simulink model "mmn_kart_candidate1_hdl"  (R2025a)
settings: Solver=FixedStepDiscrete  StartTime=0.0  StopTime=30  FixedStep=5e-5  RelTol=1e-3
undefined symbols (not defined in the file): ampa_decay, current_gain, gaba_decay, leakage_gain, refractory
libraries: simulink x3
settings Model: DataTypeOverride=Off  MinMaxOverflowLogging=MinMaxAndOverflow  FPTShortcutValueString='{{},{''BaselineRun'',1,1,1,''BaselineRun'','''',{},''M'',''SD'',''''}}'  Creator=PC  LastModifiedBy=PC
settings OptimizationCC: BlockReduction=off  ConditionallyExecuteInputs=off  DefaultParameterBehavior=Inlined
settings DebuggingCC: SingleTaskRateTransMsg=error

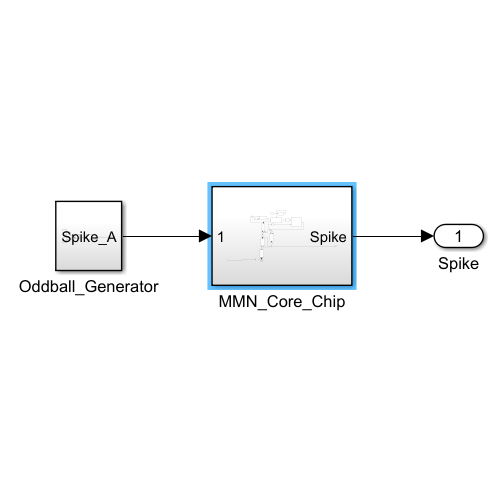
[thumbnail: Simulink's stored preview of the top-level diagram]
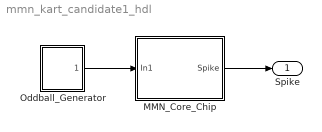
== system mmn_kart_candidate1_hdl ==
  MMN_Core_Chip : Subsystem
  Oddball_Generator : Subsystem
  Spike : Outport
  wires:
  Oddball_Generator/1(Spike_A) -> MMN_Core_Chip/1(In1)
  MMN_Core_Chip/1(Spike) -> Spike/1

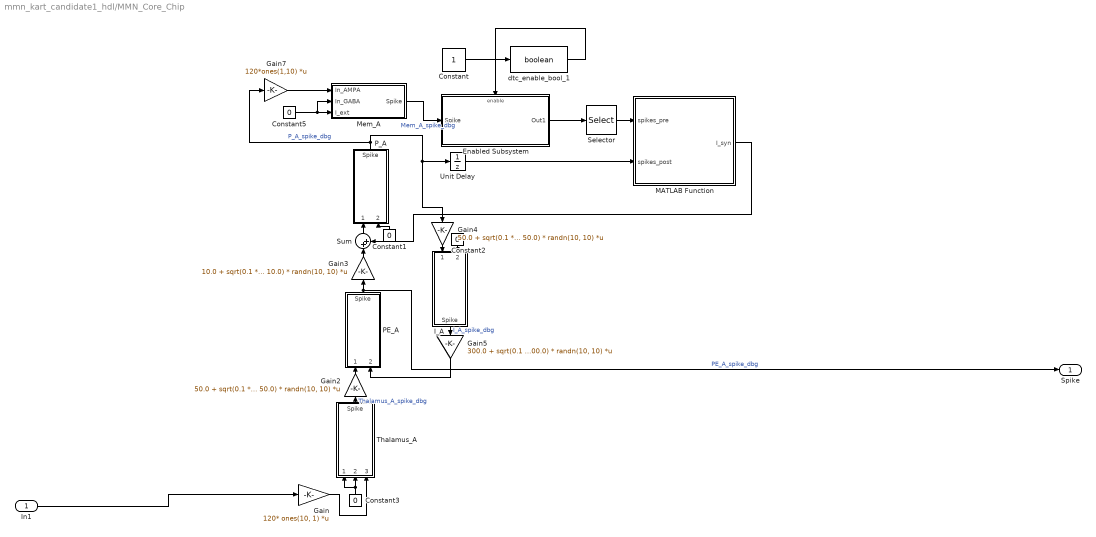
== system mmn_kart_candidate1_hdl/MMN_Core_Chip ==
  In1 : Inport  OutDataTypeStr=boolean  SampleTime=5e-5
  Constant : Constant  OutDataTypeStr=fixdt(1,24,8)  SampleTime=5e-5
  Constant{1..3,5} (4 alike) : Constant  Value=0  OutDataTypeStr=fixdt(1,24,8)
  Enabled Subsystem : Subsystem  TreatAsAtomicUnit=on
  Gain : Gain  Gain=120* ones(10, 1)  Multiplication=Matrix(K*u)  ParamDataTypeStr=fixdt(1,24,8)  OutDataTypeStr=fixdt(1,24,8)  SaturateOnIntegerOverflow=on
  Gain2 : Gain  Gain=50.0 + sqrt(0.1 * 50.0) * randn(10, 10)  Multiplication=Matrix(K*u)  ParamDataTypeStr=fixdt(1,24,8)  OutDataTypeStr=fixdt(1,24,8)  SaturateOnIntegerOverflow=on
  Gain3 : Gain  Gain=10.0 + sqrt(0.1 * 10.0) * randn(10, 10)  Multiplication=Matrix(K*u)  ParamDataTypeStr=fixdt(1,24,8)  OutDataTypeStr=fixdt(1,24,8)  SaturateOnIntegerOverflow=on
  Gain4 : Gain  Gain=50.0 + sqrt(0.1 * 50.0) * randn(10, 10)  Multiplication=Matrix(K*u)  ParamDataTypeStr=fixdt(1,24,8)  OutDataTypeStr=fixdt(1,24,8)  SaturateOnIntegerOverflow=on
  Gain5 : Gain  Gain=300.0 + sqrt(0.1 * 300.0) * randn(10, 10)  Multiplication=Matrix(K*u)  ParamDataTypeStr=fixdt(1,24,8)  OutDataTypeStr=fixdt(1,24,8)  SaturateOnIntegerOverflow=on
  Gain7 : Gain  Gain=120*ones(1,10)  Multiplication=Matrix(K*u)  ParamDataTypeStr=fixdt(1,24,8)  OutDataTypeStr=fixdt(1,24,8)  SaturateOnIntegerOverflow=on
  I_A : Subsystem
  MATLAB Function : MATLAB Function  TreatAsAtomicUnit=on  SystemSampleTime=5e-5
  Mem_A : Subsystem
  PE_A : Subsystem
  P_A : Subsystem
  Selector : Selector  InputPortWidth=12000  IndexOptions=Index vector (dialog)  Indices=[1:120:12000]  OutputSizes=1
  Sum : Sum  Inputs=|++  OutDataTypeStr=fixdt(1,24,8)  AccumDataTypeStr=fixdt(1,24,8)  SaturateOnIntegerOverflow=on
  Thalamus_A : Subsystem
  Unit Delay : UnitDelay  SampleTime=-1  HasFrameUpgradeWarning=on
  dtc_enable_bool_1 : DataTypeConversion  OutDataTypeStr=boolean  RndMeth=Floor
  Spike : Outport  OutDataTypeStr=boolean
  wires:
  Constant5/1 -> Mem_A/2("In_GABA "), Mem_A/3(I_ext)
  Sum/1 -> P_A/1(In_AMPA)
  Constant3/1 -> Thalamus_A/1(In_AMPA), Thalamus_A/2("In_GABA ")
  Constant2/1 -> I_A/2("In_GABA ")
  MATLAB Function/1(I_syn) -> Sum/2
  In1/1 -> Gain/1
  Enabled Subsystem/1(Out1) -> Selector/1
  Unit Delay/1 -> MATLAB Function/2(spikes_post)
  Mem_A/1(Spike) -> Enabled Subsystem/1(Spike)  "Mem_A_spike_dbg"
  Constant1/1 -> P_A/2("In_GABA ")
  Gain3/1 -> Sum/1
  Gain5/1 -> PE_A/2("In_GABA ")
  Gain4/1 -> I_A/1(In_AMPA)
  Gain7/1 -> Mem_A/1(In_AMPA)
  Gain2/1 -> PE_A/1(In_AMPA)
  Gain/1 -> Thalamus_A/3(I_ext)
  I_A/1(Spike) -> Gain5/1  "I_A_spike_dbg"
  Selector/1 -> MATLAB Function/1(spikes_pre)
  Thalamus_A/1(Spike) -> Gain2/1  "Thalamus_A_spike_dbg"
  PE_A/1(Spike) -> Spike/1, Gain3/1  "PE_A_spike_dbg"
  P_A/1(Spike) -> Gain4/1, Unit Delay/1, Gain7/1  "P_A_spike_dbg"
  Constant/1 -> dtc_enable_bool_1/1
  dtc_enable_bool_1/1 -> Enabled Subsystem/Enable

== system mmn_kart_candidate1_hdl/Oddball_Generator ==
  Product : Product
  Product_to_bool : DataTypeConversion  OutDataTypeStr=boolean  SaturateOnIntegerOverflow=off  RndMeth=Floor
  Pulse Generator : DiscretePulseGenerator  PulseType=Time based  Period=0.2  PulseWidth=5
  Step : Step  Time=20000  Before=1  After=0  SampleTime=5e-5
  Spike_A : Outport
  wires:
  Step/1 -> Product/2
  Pulse Generator/1 -> Product/1
  Product/1 -> Product_to_bool/1
  Product_to_bool/1 -> Spike_A/1

== system mmn_kart_candidate1_hdl/MMN_Core_Chip/Enabled Subsystem ==
  Spike : Inport
  Enable : EnablePort
  Tapped Delay : simulink/Discrete/Tapped Delay  vinit=0.0  samptime=-1  NumDelays=12000  DelayOrder=Newest  includeCurrent=off
  Out1 : Outport
  wires:
  Spike/1 -> Tapped Delay/1
  Tapped Delay/1 -> Out1/1

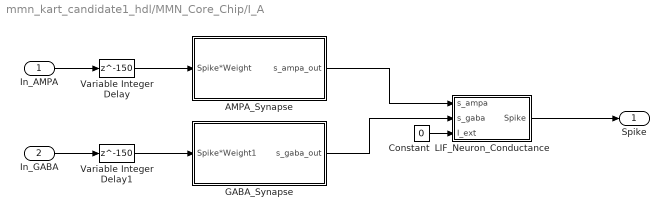
== system mmn_kart_candidate1_hdl/MMN_Core_Chip/I_A ==
  In_AMPA : Inport  OutDataTypeStr=fixdt(1,24,8)
  "In_GABA " : Inport  Port=2
  AMPA_Synapse : Subsystem
  Constant : Constant  Value=0  OutDataTypeStr=fixdt(1,24,8)
  GABA_Synapse : Subsystem
  LIF_Neuron_Conductance : Subsystem
  Variable Integer Delay : Delay  DelayLength=150
  Variable Integer Delay1 : Delay  DelayLength=150
  Spike : Outport  OutDataTypeStr=boolean
  wires:
  In_AMPA/1 -> Variable Integer Delay/1
  GABA_Synapse/1(s_gaba_out) -> LIF_Neuron_Conductance/2(s_gaba)
  LIF_Neuron_Conductance/1(Spike) -> Spike/1
  AMPA_Synapse/1(s_ampa_out) -> LIF_Neuron_Conductance/1(s_ampa)
  "In_GABA "/1 -> Variable Integer Delay1/1
  Constant/1 -> LIF_Neuron_Conductance/3(I_ext)
  Variable Integer Delay/1 -> AMPA_Synapse/1(Spike*Weight)
  Variable Integer Delay1/1 -> GABA_Synapse/1(Spike*Weight1)

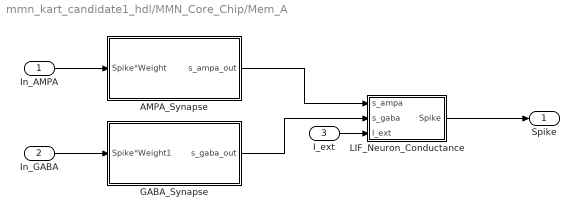
== system mmn_kart_candidate1_hdl/MMN_Core_Chip/Mem_A ==
  In_AMPA : Inport  OutDataTypeStr=fixdt(1,24,8)
  "In_GABA " : Inport  Port=2
  I_ext : Inport  Port=3  OutDataTypeStr=fixdt(1,24,8)
  AMPA_Synapse : Subsystem
  GABA_Synapse : Subsystem
  LIF_Neuron_Conductance : Subsystem
  Spike : Outport  OutDataTypeStr=boolean
  wires:
  In_AMPA/1 -> AMPA_Synapse/1(Spike*Weight)
  GABA_Synapse/1(s_gaba_out) -> LIF_Neuron_Conductance/2(s_gaba)
  LIF_Neuron_Conductance/1(Spike) -> Spike/1
  AMPA_Synapse/1(s_ampa_out) -> LIF_Neuron_Conductance/1(s_ampa)
  "In_GABA "/1 -> GABA_Synapse/1(Spike*Weight1)
  I_ext/1 -> LIF_Neuron_Conductance/3(I_ext)

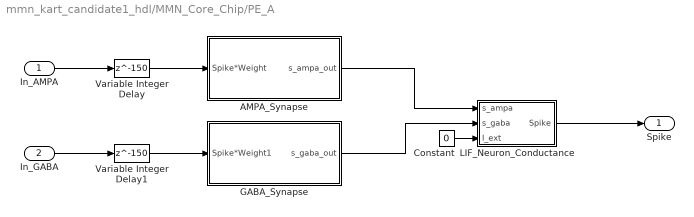
== system mmn_kart_candidate1_hdl/MMN_Core_Chip/PE_A ==
  In_AMPA : Inport  OutDataTypeStr=fixdt(1,24,8)
  "In_GABA " : Inport  Port=2
  AMPA_Synapse : Subsystem
  Constant : Constant  Value=0  OutDataTypeStr=fixdt(1,24,8)
  GABA_Synapse : Subsystem
  LIF_Neuron_Conductance : Subsystem
  Variable Integer Delay : Delay  DelayLength=150
  Variable Integer Delay1 : Delay  DelayLength=150
  Spike : Outport  OutDataTypeStr=boolean
  wires:
  In_AMPA/1 -> Variable Integer Delay/1
  GABA_Synapse/1(s_gaba_out) -> LIF_Neuron_Conductance/2(s_gaba)
  LIF_Neuron_Conductance/1(Spike) -> Spike/1
  AMPA_Synapse/1(s_ampa_out) -> LIF_Neuron_Conductance/1(s_ampa)
  "In_GABA "/1 -> Variable Integer Delay1/1
  Constant/1 -> LIF_Neuron_Conductance/3(I_ext)
  Variable Integer Delay/1 -> AMPA_Synapse/1(Spike*Weight)
  Variable Integer Delay1/1 -> GABA_Synapse/1(Spike*Weight1)

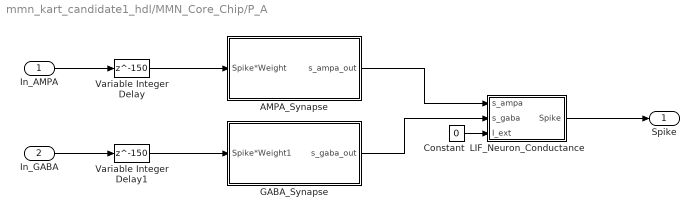
== system mmn_kart_candidate1_hdl/MMN_Core_Chip/P_A ==
  In_AMPA : Inport  OutDataTypeStr=fixdt(1,24,8)
  "In_GABA " : Inport  Port=2
  AMPA_Synapse : Subsystem
  Constant : Constant  Value=0  OutDataTypeStr=fixdt(1,24,8)
  GABA_Synapse : Subsystem
  LIF_Neuron_Conductance : Subsystem
  Variable Integer Delay : Delay  DelayLength=150
  Variable Integer Delay1 : Delay  DelayLength=150
  Spike : Outport  OutDataTypeStr=boolean
  wires:
  In_AMPA/1 -> Variable Integer Delay/1
  GABA_Synapse/1(s_gaba_out) -> LIF_Neuron_Conductance/2(s_gaba)
  LIF_Neuron_Conductance/1(Spike) -> Spike/1
  AMPA_Synapse/1(s_ampa_out) -> LIF_Neuron_Conductance/1(s_ampa)
  "In_GABA "/1 -> Variable Integer Delay1/1
  Constant/1 -> LIF_Neuron_Conductance/3(I_ext)
  Variable Integer Delay/1 -> AMPA_Synapse/1(Spike*Weight)
  Variable Integer Delay1/1 -> GABA_Synapse/1(Spike*Weight1)

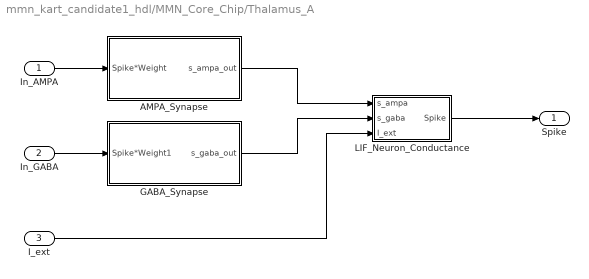
== system mmn_kart_candidate1_hdl/MMN_Core_Chip/Thalamus_A ==
  In_AMPA : Inport  OutDataTypeStr=fixdt(1,24,8)
  "In_GABA " : Inport  Port=2
  I_ext : Inport  Port=3  OutDataTypeStr=fixdt(1,24,8)
  AMPA_Synapse : Subsystem
  GABA_Synapse : Subsystem
  LIF_Neuron_Conductance : Subsystem
  Spike : Outport  OutDataTypeStr=boolean
  wires:
  In_AMPA/1 -> AMPA_Synapse/1(Spike*Weight)
  GABA_Synapse/1(s_gaba_out) -> LIF_Neuron_Conductance/2(s_gaba)
  LIF_Neuron_Conductance/1(Spike) -> Spike/1
  AMPA_Synapse/1(s_ampa_out) -> LIF_Neuron_Conductance/1(s_ampa)
  "In_GABA "/1 -> GABA_Synapse/1(Spike*Weight1)
  I_ext/1 -> LIF_Neuron_Conductance/3(I_ext)

== system mmn_kart_candidate1_hdl/MMN_Core_Chip/I_A/AMPA_Synapse ==
  Spike*Weight : Inport  OutDataTypeStr=fixdt(1,24,8)
  Add : Sum  OutDataTypeStr=fixdt(1,24,8)  AccumDataTypeStr=fixdt(1,24,8)  SaturateOnIntegerOverflow=on
  Decay_Gain : Gain  Gain=ampa_decay  ParamDataTypeStr=fixdt(1,24,20)  OutDataTypeStr=fixdt(1,24,8)  SaturateOnIntegerOverflow=on
  s_trace : UnitDelay  SampleTime=-1  HasFrameUpgradeWarning=on
  s_ampa_out : Outport  OutDataTypeStr=fixdt(1,24,8)
  wires:
  Add/1 -> s_ampa_out/1, s_trace/1
  s_trace/1 -> Decay_Gain/1
  Decay_Gain/1 -> Add/1
  Spike*Weight/1 -> Add/2

== system mmn_kart_candidate1_hdl/MMN_Core_Chip/I_A/GABA_Synapse ==
  Spike*Weight1 : Inport  OutDataTypeStr=fixdt(1,24,8)
  Add1 : Sum  OutDataTypeStr=fixdt(1,24,8)  AccumDataTypeStr=fixdt(1,24,8)  SaturateOnIntegerOverflow=on
  Decay_Gain : Gain  Gain=gaba_decay  ParamDataTypeStr=fixdt(1,24,20)  OutDataTypeStr=fixdt(1,24,8)  SaturateOnIntegerOverflow=on
  s_trace1 : UnitDelay  SampleTime=-1  HasFrameUpgradeWarning=on
  s_gaba_out : Outport  OutDataTypeStr=fixdt(1,24,8)
  wires:
  Spike*Weight1/1 -> Add1/2
  Add1/1 -> s_gaba_out/1, s_trace1/1
  s_trace1/1 -> Decay_Gain/1
  Decay_Gain/1 -> Add1/1

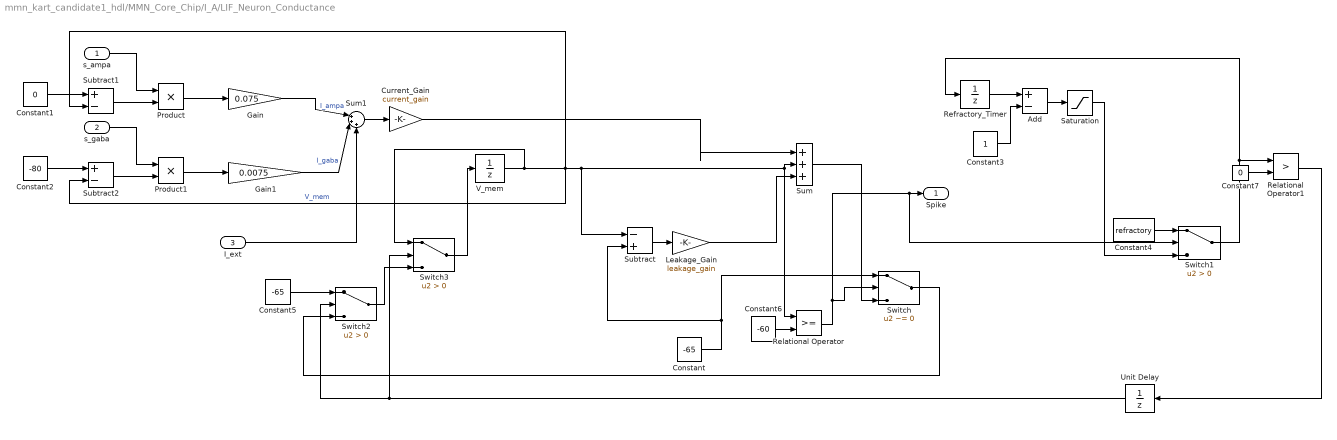
== system mmn_kart_candidate1_hdl/MMN_Core_Chip/I_A/LIF_Neuron_Conductance ==
  s_ampa : Inport  OutDataTypeStr=fixdt(1,24,8)
  s_gaba : Inport  Port=2  OutDataTypeStr=fixdt(1,24,8)
  I_ext : Inport  Port=3  OutDataTypeStr=fixdt(1,24,8)
  Add : Sum  Inputs=+-  OutDataTypeStr=fixdt(1,32,8)  AccumDataTypeStr=fixdt(1,32,8)  SaturateOnIntegerOverflow=on
  Constant : Constant  Value=-65  OutDataTypeStr=fixdt(1,32,8)
  Constant1 : Constant  Value=0  OutDataTypeStr=fixdt(1,32,8)
  Constant2 : Constant  Value=-80  OutDataTypeStr=fixdt(1,32,8)
  Constant3 : Constant  OutDataTypeStr=fixdt(1,32,8)
  Constant4 : Constant  Value=refractory  OutDataTypeStr=fixdt(1,32,8)
  Constant5 : Constant  Value=-65  OutDataTypeStr=fixdt(1,32,8)
  Constant6 : Constant  Value=-60  OutDataTypeStr=fixdt(1,32,8)
  Constant7 : Constant  Value=0  OutDataTypeStr=fixdt(1,32,8)
  Current_Gain : Gain  Gain=current_gain  ParamDataTypeStr=fixdt(1,24,20)  OutDataTypeStr=fixdt(1,32,8)  SaturateOnIntegerOverflow=on
  Gain : Gain  Gain=0.075  ParamDataTypeStr=fixdt(1,24,20)  OutDataTypeStr=fixdt(1,32,8)  SaturateOnIntegerOverflow=on
  Gain1 : Gain  Gain=0.0075  ParamDataTypeStr=fixdt(1,24,20)  OutDataTypeStr=fixdt(1,32,8)  SaturateOnIntegerOverflow=on
  Leakage_Gain : Gain  Gain=leakage_gain  ParamDataTypeStr=fixdt(1,24,20)  OutDataTypeStr=fixdt(1,32,8)  SaturateOnIntegerOverflow=on
  Product : Product  OutDataTypeStr=fixdt(1,32,8)  SaturateOnIntegerOverflow=on
  Product1 : Product  OutDataTypeStr=fixdt(1,32,8)  SaturateOnIntegerOverflow=on
  Refractory_Timer : UnitDelay  SampleTime=-1  HasFrameUpgradeWarning=on
  Relational Operator : RelationalOperator  OutDataTypeStr=boolean  RndMeth=Simplest  InputSameDT=off
  Relational Operator1 : RelationalOperator  Operator=>  OutDataTypeStr=boolean  RndMeth=Simplest  InputSameDT=off
  Saturation : Saturate  UpperLimit=40  LowerLimit=0  OutDataTypeStr=fixdt(1,32,8)
  Subtract : Sum  Inputs=-+  OutDataTypeStr=fixdt(1,32,8)  AccumDataTypeStr=fixdt(1,32,8)  SaturateOnIntegerOverflow=on
  Subtract1 : Sum  Inputs=+-  OutDataTypeStr=fixdt(1,32,8)  AccumDataTypeStr=fixdt(1,32,8)  SaturateOnIntegerOverflow=on
  Subtract2 : Sum  Inputs=+-  OutDataTypeStr=fixdt(1,32,8)  AccumDataTypeStr=fixdt(1,32,8)  SaturateOnIntegerOverflow=on
  Sum : Sum  Inputs=|+++  OutDataTypeStr=fixdt(1,32,8)  AccumDataTypeStr=fixdt(1,32,8)  SaturateOnIntegerOverflow=on
  Sum1 : Sum  Inputs=|+++  OutDataTypeStr=fixdt(1,32,8)  AccumDataTypeStr=fixdt(1,32,8)  SaturateOnIntegerOverflow=on
  Switch : Switch  Criteria=u2 ~= 0  OutDataTypeStr=fixdt(1,32,8)  InputSameDT=off
  Switch1 : Switch  Criteria=u2 > Threshold  OutDataTypeStr=fixdt(1,32,8)  InputSameDT=off
  Switch2 : Switch  Criteria=u2 > Threshold  OutDataTypeStr=fixdt(1,32,8)  InputSameDT=off
  Switch3 : Switch  Criteria=u2 > Threshold  OutDataTypeStr=fixdt(1,32,8)  InputSameDT=off
  Unit Delay : UnitDelay  SampleTime=-1  HasFrameUpgradeWarning=on
  V_mem : UnitDelay  InitialCondition=-65* ones(10, 1)  SampleTime=-1  HasFrameUpgradeWarning=on
  Spike : Outport  OutDataTypeStr=boolean
  wires:
  Gain1/1 -> Sum1/2  "I_gaba"
  Leakage_Gain/1 -> Sum/3
  Subtract2/1 -> Product1/2
  Relational Operator/1 -> Switch1/2, Spike/1, Switch/2
  Constant1/1 -> Subtract1/1
  Constant/1 -> Subtract/2, Switch/1
  s_ampa/1 -> Product/1
  Product/1 -> Gain/1
  Subtract1/1 -> Product/2
  Gain/1 -> Sum1/1  "I_ampa"
  Switch/1 -> Switch2/3
  Product1/1 -> Gain1/1
  s_gaba/1 -> Product1/1
  Subtract/1 -> Leakage_Gain/1
  Constant2/1 -> Subtract2/1
  Current_Gain/1 -> Sum/1
  Sum/1 -> Switch/3
  Sum1/1 -> Current_Gain/1
  I_ext/1 -> Sum1/3
  Refractory_Timer/1 -> Add/1
  Constant3/1 -> Add/2
  Add/1 -> Saturation/1
  Constant4/1 -> Switch1/1
  Saturation/1 -> Switch1/3
  Switch1/1 -> Refractory_Timer/1, Relational Operator1/1
  Relational Operator1/1 -> Unit Delay/1
  Constant5/1 -> Switch2/1
  Constant6/1 -> Relational Operator/2
  Constant7/1 -> Relational Operator1/2
  Unit Delay/1 -> Switch3/2, Switch2/2
  V_mem/1 -> Subtract1/2, Subtract2/2, Relational Operator/1, Sum/2, Subtract/1, Switch3/1  "V_mem"
  Switch2/1 -> Switch3/3
  Switch3/1 -> V_mem/1

== system mmn_kart_candidate1_hdl/MMN_Core_Chip/Mem_A/AMPA_Synapse ==
  Spike*Weight : Inport  OutDataTypeStr=fixdt(1,24,8)
  Add : Sum  OutDataTypeStr=fixdt(1,24,8)  AccumDataTypeStr=fixdt(1,24,8)  SaturateOnIntegerOverflow=on
  Decay_Gain : Gain  Gain=ampa_decay  ParamDataTypeStr=fixdt(1,24,20)  OutDataTypeStr=fixdt(1,24,8)  SaturateOnIntegerOverflow=on
  s_trace : UnitDelay  SampleTime=-1  HasFrameUpgradeWarning=on
  s_ampa_out : Outport  OutDataTypeStr=fixdt(1,24,8)
  wires:
  Add/1 -> s_ampa_out/1, s_trace/1
  s_trace/1 -> Decay_Gain/1
  Decay_Gain/1 -> Add/1
  Spike*Weight/1 -> Add/2

== system mmn_kart_candidate1_hdl/MMN_Core_Chip/Mem_A/GABA_Synapse ==
  Spike*Weight1 : Inport  OutDataTypeStr=fixdt(1,24,8)
  Add1 : Sum  OutDataTypeStr=fixdt(1,24,8)  AccumDataTypeStr=fixdt(1,24,8)  SaturateOnIntegerOverflow=on
  Decay_Gain : Gain  Gain=gaba_decay  ParamDataTypeStr=fixdt(1,24,20)  OutDataTypeStr=fixdt(1,24,8)  SaturateOnIntegerOverflow=on
  s_trace1 : UnitDelay  SampleTime=-1  HasFrameUpgradeWarning=on
  s_gaba_out : Outport  OutDataTypeStr=fixdt(1,24,8)
  wires:
  Spike*Weight1/1 -> Add1/2
  Add1/1 -> s_gaba_out/1, s_trace1/1
  s_trace1/1 -> Decay_Gain/1
  Decay_Gain/1 -> Add1/1

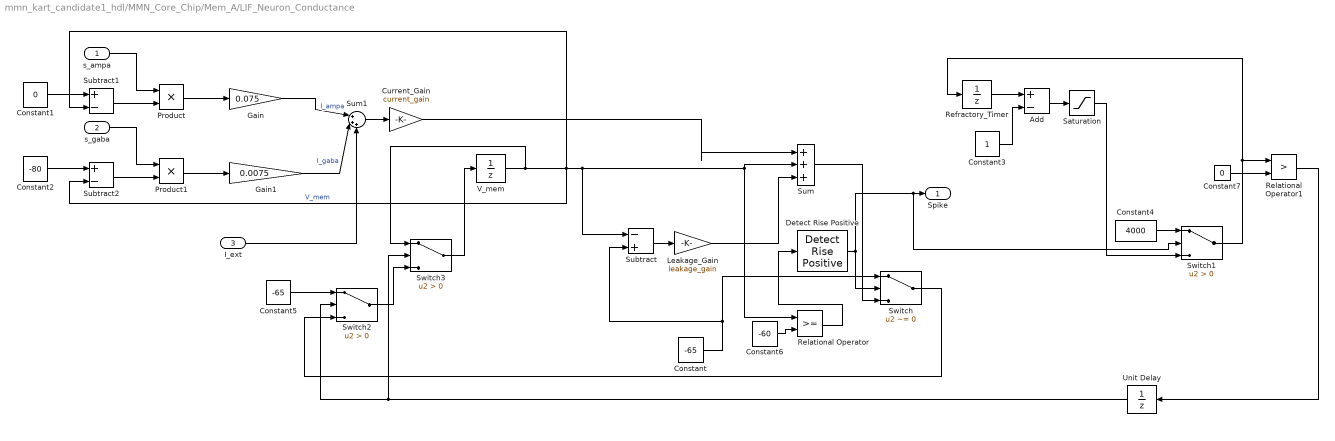
== system mmn_kart_candidate1_hdl/MMN_Core_Chip/Mem_A/LIF_Neuron_Conductance ==
  s_ampa : Inport  OutDataTypeStr=fixdt(1,24,8)
  s_gaba : Inport  Port=2  OutDataTypeStr=fixdt(1,24,8)
  I_ext : Inport  Port=3  OutDataTypeStr=fixdt(1,24,8)
  Add : Sum  Inputs=+-  OutDataTypeStr=fixdt(1,32,8)  AccumDataTypeStr=fixdt(1,32,8)  SaturateOnIntegerOverflow=on
  Constant : Constant  Value=-65  OutDataTypeStr=fixdt(1,32,8)
  Constant1 : Constant  Value=0  OutDataTypeStr=fixdt(1,32,8)
  Constant2 : Constant  Value=-80  OutDataTypeStr=fixdt(1,32,8)
  Constant3 : Constant  OutDataTypeStr=fixdt(1,32,8)
  Constant4 : Constant  Value=4000  OutDataTypeStr=fixdt(1,32,8)
  Constant5 : Constant  Value=-65  OutDataTypeStr=fixdt(1,32,8)
  Constant6 : Constant  Value=-60  OutDataTypeStr=fixdt(1,32,8)
  Constant7 : Constant  Value=0  OutDataTypeStr=fixdt(1,32,8)
  Current_Gain : Gain  Gain=current_gain  ParamDataTypeStr=fixdt(1,24,20)  OutDataTypeStr=fixdt(1,32,8)  SaturateOnIntegerOverflow=on
  Detect Rise Positive : simulink/Logic and Bit Operations/Detect Rise Positive  vinit=0  OutDataTypeStr=boolean
      link override FixPt Relational Operator: OutDataTypeStr=boolean
      link override Positive/Compare: OutDataTypeStr=boolean
      link override Positive/Constant: OutDataTypeStr=boolean
      link override Positive/u: OutDataTypeStr=boolean
      link override Positive/y: OutDataTypeStr=boolean
      link override U: OutDataTypeStr=boolean
      link override Y: OutDataTypeStr=boolean
  Gain : Gain  Gain=0.075  ParamDataTypeStr=fixdt(1,24,20)  OutDataTypeStr=fixdt(1,32,8)  SaturateOnIntegerOverflow=on
  Gain1 : Gain  Gain=0.0075  ParamDataTypeStr=fixdt(1,24,20)  OutDataTypeStr=fixdt(1,32,8)  SaturateOnIntegerOverflow=on
  Leakage_Gain : Gain  Gain=leakage_gain  ParamDataTypeStr=fixdt(1,24,20)  OutDataTypeStr=fixdt(1,32,8)  SaturateOnIntegerOverflow=on
  Product : Product  OutDataTypeStr=fixdt(1,32,8)  SaturateOnIntegerOverflow=on
  Product1 : Product  OutDataTypeStr=fixdt(1,32,8)  SaturateOnIntegerOverflow=on
  Refractory_Timer : UnitDelay  SampleTime=-1  HasFrameUpgradeWarning=on
  Relational Operator : RelationalOperator  OutDataTypeStr=boolean  RndMeth=Simplest  InputSameDT=off
  Relational Operator1 : RelationalOperator  Operator=>  OutDataTypeStr=boolean  RndMeth=Simplest  InputSameDT=off
  Saturation : Saturate  UpperLimit=4000  LowerLimit=0  OutDataTypeStr=fixdt(1,32,8)
  Subtract : Sum  Inputs=-+  OutDataTypeStr=fixdt(1,32,8)  AccumDataTypeStr=fixdt(1,32,8)  SaturateOnIntegerOverflow=on
  Subtract1 : Sum  Inputs=+-  OutDataTypeStr=fixdt(1,32,8)  AccumDataTypeStr=fixdt(1,32,8)  SaturateOnIntegerOverflow=on
  Subtract2 : Sum  Inputs=+-  OutDataTypeStr=fixdt(1,32,8)  AccumDataTypeStr=fixdt(1,32,8)  SaturateOnIntegerOverflow=on
  Sum : Sum  Inputs=|+++  OutDataTypeStr=fixdt(1,32,8)  AccumDataTypeStr=fixdt(1,32,8)  SaturateOnIntegerOverflow=on
  Sum1 : Sum  Inputs=|+++  OutDataTypeStr=fixdt(1,32,8)  AccumDataTypeStr=fixdt(1,32,8)  SaturateOnIntegerOverflow=on
  Switch : Switch  Criteria=u2 ~= 0  OutDataTypeStr=fixdt(1,32,8)  InputSameDT=off
  Switch1 : Switch  Criteria=u2 > Threshold  OutDataTypeStr=fixdt(1,32,8)  InputSameDT=off
  Switch2 : Switch  Criteria=u2 > Threshold  OutDataTypeStr=fixdt(1,32,8)  InputSameDT=off
  Switch3 : Switch  Criteria=u2 > Threshold  OutDataTypeStr=fixdt(1,32,8)  InputSameDT=off
  Unit Delay : UnitDelay  SampleTime=-1  HasFrameUpgradeWarning=on
  V_mem : UnitDelay  InitialCondition=-65  SampleTime=-1  HasFrameUpgradeWarning=on
  Spike : Outport  OutDataTypeStr=boolean
  wires:
  Gain1/1 -> Sum1/2  "I_gaba"
  V_mem/1 -> Switch3/1, Subtract1/2, Subtract2/2, Relational Operator/1, Sum/2, Subtract/1  "V_mem"
  Leakage_Gain/1 -> Sum/3
  Subtract2/1 -> Product1/2
  Constant1/1 -> Subtract1/1
  Constant/1 -> Subtract/2, Switch/1
  s_ampa/1 -> Product/1
  Product/1 -> Gain/1
  Subtract1/1 -> Product/2
  Gain/1 -> Sum1/1  "I_ampa"
  Switch/1 -> Switch2/3
  Product1/1 -> Gain1/1
  s_gaba/1 -> Product1/1
  Subtract/1 -> Leakage_Gain/1
  Constant2/1 -> Subtract2/1
  Current_Gain/1 -> Sum/1
  Sum/1 -> Switch/3
  Sum1/1 -> Current_Gain/1
  I_ext/1 -> Sum1/3
  Refractory_Timer/1 -> Add/1
  Constant3/1 -> Add/2
  Add/1 -> Saturation/1
  Constant4/1 -> Switch1/1
  Saturation/1 -> Switch1/3
  Switch1/1 -> Refractory_Timer/1, Relational Operator1/1
  Relational Operator1/1 -> Unit Delay/1
  Constant5/1 -> Switch2/1
  Switch2/1 -> Switch3/3
  Unit Delay/1 -> Switch3/2, Switch2/2
  Constant6/1 -> Relational Operator/2
  Constant7/1 -> Relational Operator1/2
  Switch3/1 -> V_mem/1
  Relational Operator/1 -> Detect Rise Positive/1
  Detect Rise Positive/1 -> Switch1/2, Spike/1, Switch/2

== system mmn_kart_candidate1_hdl/MMN_Core_Chip/PE_A/AMPA_Synapse ==
  Spike*Weight : Inport  OutDataTypeStr=fixdt(1,24,8)
  Add : Sum  OutDataTypeStr=fixdt(1,24,8)  AccumDataTypeStr=fixdt(1,24,8)  SaturateOnIntegerOverflow=on
  Decay_Gain : Gain  Gain=ampa_decay  ParamDataTypeStr=fixdt(1,24,20)  OutDataTypeStr=fixdt(1,24,8)  SaturateOnIntegerOverflow=on
  s_trace : UnitDelay  SampleTime=-1  HasFrameUpgradeWarning=on
  s_ampa_out : Outport  OutDataTypeStr=fixdt(1,24,8)
  wires:
  Add/1 -> s_ampa_out/1, s_trace/1
  s_trace/1 -> Decay_Gain/1
  Decay_Gain/1 -> Add/1
  Spike*Weight/1 -> Add/2

== system mmn_kart_candidate1_hdl/MMN_Core_Chip/PE_A/GABA_Synapse ==
  Spike*Weight1 : Inport  OutDataTypeStr=fixdt(1,24,8)
  Add1 : Sum  OutDataTypeStr=fixdt(1,24,8)  AccumDataTypeStr=fixdt(1,24,8)  SaturateOnIntegerOverflow=on
  Decay_Gain : Gain  Gain=gaba_decay  ParamDataTypeStr=fixdt(1,24,20)  OutDataTypeStr=fixdt(1,24,8)  SaturateOnIntegerOverflow=on
  s_trace1 : UnitDelay  SampleTime=-1  HasFrameUpgradeWarning=on
  s_gaba_out : Outport  OutDataTypeStr=fixdt(1,24,8)
  wires:
  Spike*Weight1/1 -> Add1/2
  Add1/1 -> s_gaba_out/1, s_trace1/1
  s_trace1/1 -> Decay_Gain/1
  Decay_Gain/1 -> Add1/1

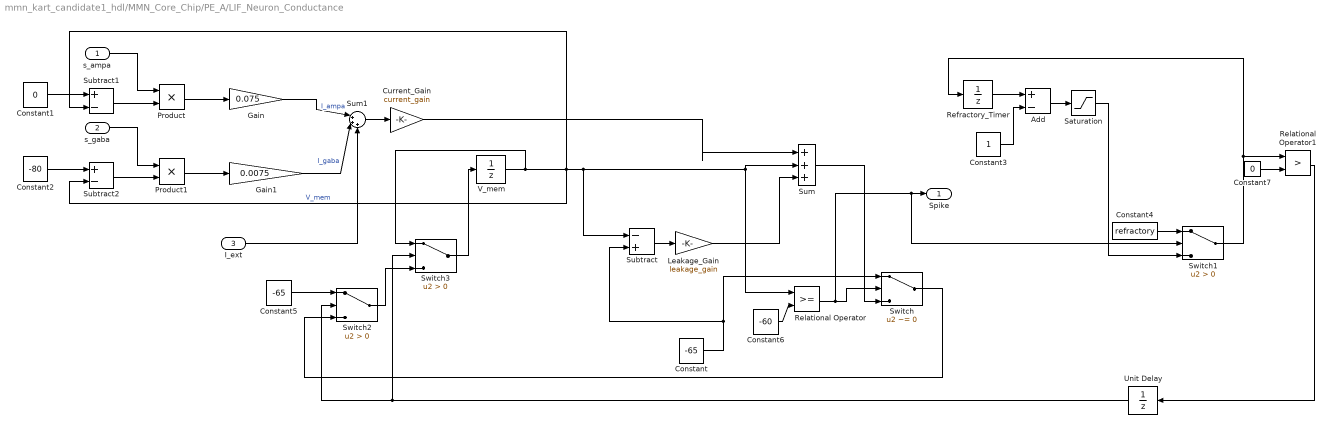
== system mmn_kart_candidate1_hdl/MMN_Core_Chip/PE_A/LIF_Neuron_Conductance ==
  s_ampa : Inport  OutDataTypeStr=fixdt(1,24,8)
  s_gaba : Inport  Port=2  OutDataTypeStr=fixdt(1,24,8)
  I_ext : Inport  Port=3  OutDataTypeStr=fixdt(1,24,8)
  Add : Sum  Inputs=+-  OutDataTypeStr=fixdt(1,32,8)  AccumDataTypeStr=fixdt(1,32,8)  SaturateOnIntegerOverflow=on
  Constant : Constant  Value=-65  OutDataTypeStr=fixdt(1,32,8)
  Constant1 : Constant  Value=0  OutDataTypeStr=fixdt(1,32,8)
  Constant2 : Constant  Value=-80  OutDataTypeStr=fixdt(1,32,8)
  Constant3 : Constant  OutDataTypeStr=fixdt(1,32,8)
  Constant4 : Constant  Value=refractory  OutDataTypeStr=fixdt(1,32,8)
  Constant5 : Constant  Value=-65  OutDataTypeStr=fixdt(1,32,8)
  Constant6 : Constant  Value=-60  OutDataTypeStr=fixdt(1,32,8)
  Constant7 : Constant  Value=0  OutDataTypeStr=fixdt(1,32,8)
  Current_Gain : Gain  Gain=current_gain  ParamDataTypeStr=fixdt(1,24,20)  OutDataTypeStr=fixdt(1,32,8)  SaturateOnIntegerOverflow=on
  Gain : Gain  Gain=0.075  ParamDataTypeStr=fixdt(1,24,20)  OutDataTypeStr=fixdt(1,32,8)  SaturateOnIntegerOverflow=on
  Gain1 : Gain  Gain=0.0075  ParamDataTypeStr=fixdt(1,24,20)  OutDataTypeStr=fixdt(1,32,8)  SaturateOnIntegerOverflow=on
  Leakage_Gain : Gain  Gain=leakage_gain  ParamDataTypeStr=fixdt(1,24,20)  OutDataTypeStr=fixdt(1,32,8)  SaturateOnIntegerOverflow=on
  Product : Product  OutDataTypeStr=fixdt(1,32,8)  SaturateOnIntegerOverflow=on
  Product1 : Product  OutDataTypeStr=fixdt(1,32,8)  SaturateOnIntegerOverflow=on
  Refractory_Timer : UnitDelay  SampleTime=-1  HasFrameUpgradeWarning=on
  Relational Operator : RelationalOperator  OutDataTypeStr=boolean  RndMeth=Simplest  InputSameDT=off
  Relational Operator1 : RelationalOperator  Operator=>  OutDataTypeStr=boolean  RndMeth=Simplest  InputSameDT=off
  Saturation : Saturate  UpperLimit=40  LowerLimit=0  OutDataTypeStr=fixdt(1,32,8)
  Subtract : Sum  Inputs=-+  OutDataTypeStr=fixdt(1,32,8)  AccumDataTypeStr=fixdt(1,32,8)  SaturateOnIntegerOverflow=on
  Subtract1 : Sum  Inputs=+-  OutDataTypeStr=fixdt(1,32,8)  AccumDataTypeStr=fixdt(1,32,8)  SaturateOnIntegerOverflow=on
  Subtract2 : Sum  Inputs=+-  OutDataTypeStr=fixdt(1,32,8)  AccumDataTypeStr=fixdt(1,32,8)  SaturateOnIntegerOverflow=on
  Sum : Sum  Inputs=|+++  OutDataTypeStr=fixdt(1,32,8)  AccumDataTypeStr=fixdt(1,32,8)  SaturateOnIntegerOverflow=on
  Sum1 : Sum  Inputs=|+++  OutDataTypeStr=fixdt(1,32,8)  AccumDataTypeStr=fixdt(1,32,8)  SaturateOnIntegerOverflow=on
  Switch : Switch  Criteria=u2 ~= 0  OutDataTypeStr=fixdt(1,32,8)  InputSameDT=off
  Switch1 : Switch  Criteria=u2 > Threshold  OutDataTypeStr=fixdt(1,32,8)  InputSameDT=off
  Switch2 : Switch  Criteria=u2 > Threshold  OutDataTypeStr=fixdt(1,32,8)  InputSameDT=off
  Switch3 : Switch  Criteria=u2 > Threshold  OutDataTypeStr=fixdt(1,32,8)  InputSameDT=off
  Unit Delay : UnitDelay  SampleTime=-1  HasFrameUpgradeWarning=on
  V_mem : UnitDelay  InitialCondition=-65* ones(10, 1)  SampleTime=-1  HasFrameUpgradeWarning=on
  Spike : Outport  OutDataTypeStr=boolean
  wires:
  Gain1/1 -> Sum1/2  "I_gaba"
  Leakage_Gain/1 -> Sum/3
  Subtract2/1 -> Product1/2
  Relational Operator/1 -> Switch1/2, Spike/1, Switch/2
  Constant1/1 -> Subtract1/1
  Constant/1 -> Subtract/2, Switch/1
  s_ampa/1 -> Product/1
  Product/1 -> Gain/1
  Subtract1/1 -> Product/2
  Gain/1 -> Sum1/1  "I_ampa"
  Switch/1 -> Switch2/3
  Product1/1 -> Gain1/1
  s_gaba/1 -> Product1/1
  Subtract/1 -> Leakage_Gain/1
  Constant2/1 -> Subtract2/1
  Current_Gain/1 -> Sum/1
  Sum/1 -> Switch/3
  Sum1/1 -> Current_Gain/1
  I_ext/1 -> Sum1/3
  Refractory_Timer/1 -> Add/1
  Constant3/1 -> Add/2
  Add/1 -> Saturation/1
  Constant4/1 -> Switch1/1
  Saturation/1 -> Switch1/3
  Switch1/1 -> Refractory_Timer/1, Relational Operator1/1
  Relational Operator1/1 -> Unit Delay/1
  Constant5/1 -> Switch2/1
  Constant6/1 -> Relational Operator/2
  Constant7/1 -> Relational Operator1/2
  Unit Delay/1 -> Switch3/2, Switch2/2
  V_mem/1 -> Subtract1/2, Subtract2/2, Relational Operator/1, Sum/2, Subtract/1, Switch3/1  "V_mem"
  Switch2/1 -> Switch3/3
  Switch3/1 -> V_mem/1

== system mmn_kart_candidate1_hdl/MMN_Core_Chip/P_A/AMPA_Synapse ==
  Spike*Weight : Inport  OutDataTypeStr=fixdt(1,24,8)
  Add : Sum  OutDataTypeStr=fixdt(1,24,8)  AccumDataTypeStr=fixdt(1,24,8)  SaturateOnIntegerOverflow=on
  Decay_Gain : Gain  Gain=ampa_decay  ParamDataTypeStr=fixdt(1,24,20)  OutDataTypeStr=fixdt(1,24,8)  SaturateOnIntegerOverflow=on
  s_trace : UnitDelay  SampleTime=-1  HasFrameUpgradeWarning=on
  s_ampa_out : Outport  OutDataTypeStr=fixdt(1,24,8)
  wires:
  Add/1 -> s_ampa_out/1, s_trace/1
  s_trace/1 -> Decay_Gain/1
  Decay_Gain/1 -> Add/1
  Spike*Weight/1 -> Add/2

== system mmn_kart_candidate1_hdl/MMN_Core_Chip/P_A/GABA_Synapse ==
  Spike*Weight1 : Inport  OutDataTypeStr=fixdt(1,24,8)
  Add1 : Sum  OutDataTypeStr=fixdt(1,24,8)  AccumDataTypeStr=fixdt(1,24,8)  SaturateOnIntegerOverflow=on
  Decay_Gain : Gain  Gain=gaba_decay  ParamDataTypeStr=fixdt(1,24,20)  OutDataTypeStr=fixdt(1,24,8)  SaturateOnIntegerOverflow=on
  s_trace1 : UnitDelay  SampleTime=-1  HasFrameUpgradeWarning=on
  s_gaba_out : Outport  OutDataTypeStr=fixdt(1,24,8)
  wires:
  Spike*Weight1/1 -> Add1/2
  Add1/1 -> s_gaba_out/1, s_trace1/1
  s_trace1/1 -> Decay_Gain/1
  Decay_Gain/1 -> Add1/1

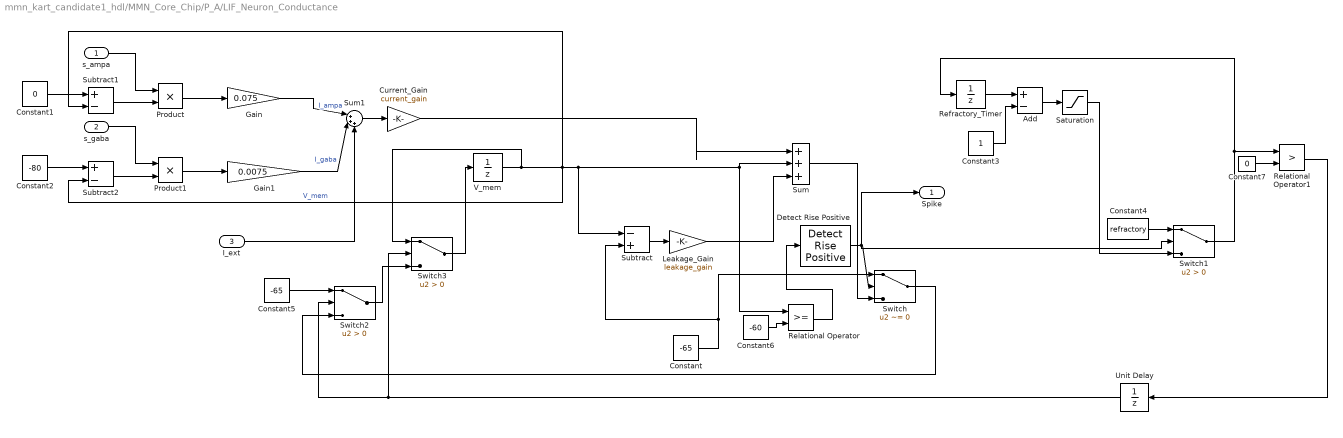
== system mmn_kart_candidate1_hdl/MMN_Core_Chip/P_A/LIF_Neuron_Conductance ==
  s_ampa : Inport  OutDataTypeStr=fixdt(1,24,8)
  s_gaba : Inport  Port=2  OutDataTypeStr=fixdt(1,24,8)
  I_ext : Inport  Port=3  OutDataTypeStr=fixdt(1,24,8)
  Add : Sum  Inputs=+-  OutDataTypeStr=fixdt(1,32,8)  AccumDataTypeStr=fixdt(1,32,8)  SaturateOnIntegerOverflow=on
  Constant : Constant  Value=-65  OutDataTypeStr=fixdt(1,32,8)
  Constant1 : Constant  Value=0  OutDataTypeStr=fixdt(1,32,8)
  Constant2 : Constant  Value=-80  OutDataTypeStr=fixdt(1,32,8)
  Constant3 : Constant  OutDataTypeStr=fixdt(1,32,8)
  Constant4 : Constant  Value=refractory  OutDataTypeStr=fixdt(1,32,8)
  Constant5 : Constant  Value=-65  OutDataTypeStr=fixdt(1,32,8)
  Constant6 : Constant  Value=-60  OutDataTypeStr=fixdt(1,32,8)
  Constant7 : Constant  Value=0  OutDataTypeStr=fixdt(1,32,8)
  Current_Gain : Gain  Gain=current_gain  ParamDataTypeStr=fixdt(1,24,20)  OutDataTypeStr=fixdt(1,32,8)  SaturateOnIntegerOverflow=on
  Detect Rise Positive : simulink/Logic and Bit Operations/Detect Rise Positive  vinit=0  OutDataTypeStr=boolean
      link override FixPt Relational Operator: OutDataTypeStr=boolean
      link override Positive/Compare: OutDataTypeStr=boolean
      link override Positive/Constant: OutDataTypeStr=boolean
      link override Positive/u: OutDataTypeStr=boolean
      link override Positive/y: OutDataTypeStr=boolean
      link override U: OutDataTypeStr=boolean
      link override Y: OutDataTypeStr=boolean
  Gain : Gain  Gain=0.075  ParamDataTypeStr=fixdt(1,24,20)  OutDataTypeStr=fixdt(1,32,8)  SaturateOnIntegerOverflow=on
  Gain1 : Gain  Gain=0.0075  ParamDataTypeStr=fixdt(1,24,20)  OutDataTypeStr=fixdt(1,32,8)  SaturateOnIntegerOverflow=on
  Leakage_Gain : Gain  Gain=leakage_gain  ParamDataTypeStr=fixdt(1,24,20)  OutDataTypeStr=fixdt(1,32,8)  SaturateOnIntegerOverflow=on
  Product : Product  OutDataTypeStr=fixdt(1,32,8)  SaturateOnIntegerOverflow=on
  Product1 : Product  OutDataTypeStr=fixdt(1,32,8)  SaturateOnIntegerOverflow=on
  Refractory_Timer : UnitDelay  SampleTime=-1  HasFrameUpgradeWarning=on
  Relational Operator : RelationalOperator  OutDataTypeStr=boolean  RndMeth=Simplest  InputSameDT=off
  Relational Operator1 : RelationalOperator  Operator=>  OutDataTypeStr=boolean  RndMeth=Simplest  InputSameDT=off
  Saturation : Saturate  UpperLimit=40  LowerLimit=0  OutDataTypeStr=fixdt(1,32,8)
  Subtract : Sum  Inputs=-+  OutDataTypeStr=fixdt(1,32,8)  AccumDataTypeStr=fixdt(1,32,8)  SaturateOnIntegerOverflow=on
  Subtract1 : Sum  Inputs=+-  OutDataTypeStr=fixdt(1,32,8)  AccumDataTypeStr=fixdt(1,32,8)  SaturateOnIntegerOverflow=on
  Subtract2 : Sum  Inputs=+-  OutDataTypeStr=fixdt(1,32,8)  AccumDataTypeStr=fixdt(1,32,8)  SaturateOnIntegerOverflow=on
  Sum : Sum  Inputs=|+++  OutDataTypeStr=fixdt(1,32,8)  AccumDataTypeStr=fixdt(1,32,8)  SaturateOnIntegerOverflow=on
  Sum1 : Sum  Inputs=|+++  OutDataTypeStr=fixdt(1,32,8)  AccumDataTypeStr=fixdt(1,32,8)  SaturateOnIntegerOverflow=on
  Switch : Switch  Criteria=u2 ~= 0  OutDataTypeStr=fixdt(1,32,8)  InputSameDT=off
  Switch1 : Switch  Criteria=u2 > Threshold  OutDataTypeStr=fixdt(1,32,8)  InputSameDT=off
  Switch2 : Switch  Criteria=u2 > Threshold  OutDataTypeStr=fixdt(1,32,8)  InputSameDT=off
  Switch3 : Switch  Criteria=u2 > Threshold  OutDataTypeStr=fixdt(1,32,8)  InputSameDT=off
  Unit Delay : UnitDelay  SampleTime=-1  HasFrameUpgradeWarning=on
  V_mem : UnitDelay  InitialCondition=-65* ones(10, 1)  SampleTime=-1  HasFrameUpgradeWarning=on
  Spike : Outport  OutDataTypeStr=boolean
  wires:
  Gain1/1 -> Sum1/2  "I_gaba"
  Leakage_Gain/1 -> Sum/3
  Subtract2/1 -> Product1/2
  Constant1/1 -> Subtract1/1
  Constant/1 -> Subtract/2, Switch/1
  s_ampa/1 -> Product/1
  Product/1 -> Gain/1
  Subtract1/1 -> Product/2
  Gain/1 -> Sum1/1  "I_ampa"
  Switch/1 -> Switch2/3
  Product1/1 -> Gain1/1
  s_gaba/1 -> Product1/1
  Subtract/1 -> Leakage_Gain/1
  Constant2/1 -> Subtract2/1
  Current_Gain/1 -> Sum/1
  Sum/1 -> Switch/3
  Sum1/1 -> Current_Gain/1
  I_ext/1 -> Sum1/3
  Refractory_Timer/1 -> Add/1
  Constant3/1 -> Add/2
  Add/1 -> Saturation/1
  Constant4/1 -> Switch1/1
  Saturation/1 -> Switch1/3
  Switch1/1 -> Refractory_Timer/1, Relational Operator1/1
  Relational Operator1/1 -> Unit Delay/1
  Constant5/1 -> Switch2/1
  Constant6/1 -> Relational Operator/2
  Constant7/1 -> Relational Operator1/2
  Unit Delay/1 -> Switch3/2, Switch2/2
  V_mem/1 -> Subtract1/2, Subtract2/2, Relational Operator/1, Sum/2, Subtract/1, Switch3/1  "V_mem"
  Switch2/1 -> Switch3/3
  Switch3/1 -> V_mem/1
  Detect Rise Positive/1 -> Spike/1, Switch1/2, Switch/2
  Relational Operator/1 -> Detect Rise Positive/1

== system mmn_kart_candidate1_hdl/MMN_Core_Chip/Thalamus_A/AMPA_Synapse ==
  Spike*Weight : Inport  OutDataTypeStr=fixdt(1,24,8)
  Add : Sum  OutDataTypeStr=fixdt(1,24,8)  AccumDataTypeStr=fixdt(1,24,8)  SaturateOnIntegerOverflow=on
  Decay_Gain : Gain  Gain=ampa_decay  ParamDataTypeStr=fixdt(1,24,20)  OutDataTypeStr=fixdt(1,24,8)  SaturateOnIntegerOverflow=on
  s_trace : UnitDelay  SampleTime=-1  HasFrameUpgradeWarning=on
  s_ampa_out : Outport  OutDataTypeStr=fixdt(1,24,8)
  wires:
  Add/1 -> s_ampa_out/1, s_trace/1
  s_trace/1 -> Decay_Gain/1
  Decay_Gain/1 -> Add/1
  Spike*Weight/1 -> Add/2

== system mmn_kart_candidate1_hdl/MMN_Core_Chip/Thalamus_A/GABA_Synapse ==
  Spike*Weight1 : Inport  OutDataTypeStr=fixdt(1,24,8)
  Add1 : Sum  OutDataTypeStr=fixdt(1,24,8)  AccumDataTypeStr=fixdt(1,24,8)  SaturateOnIntegerOverflow=on
  Decay_Gain : Gain  Gain=gaba_decay  ParamDataTypeStr=fixdt(1,24,20)  OutDataTypeStr=fixdt(1,24,8)  SaturateOnIntegerOverflow=on
  s_trace1 : UnitDelay  SampleTime=-1  HasFrameUpgradeWarning=on
  s_gaba_out : Outport  OutDataTypeStr=fixdt(1,24,8)
  wires:
  Spike*Weight1/1 -> Add1/2
  Add1/1 -> s_gaba_out/1, s_trace1/1
  s_trace1/1 -> Decay_Gain/1
  Decay_Gain/1 -> Add1/1

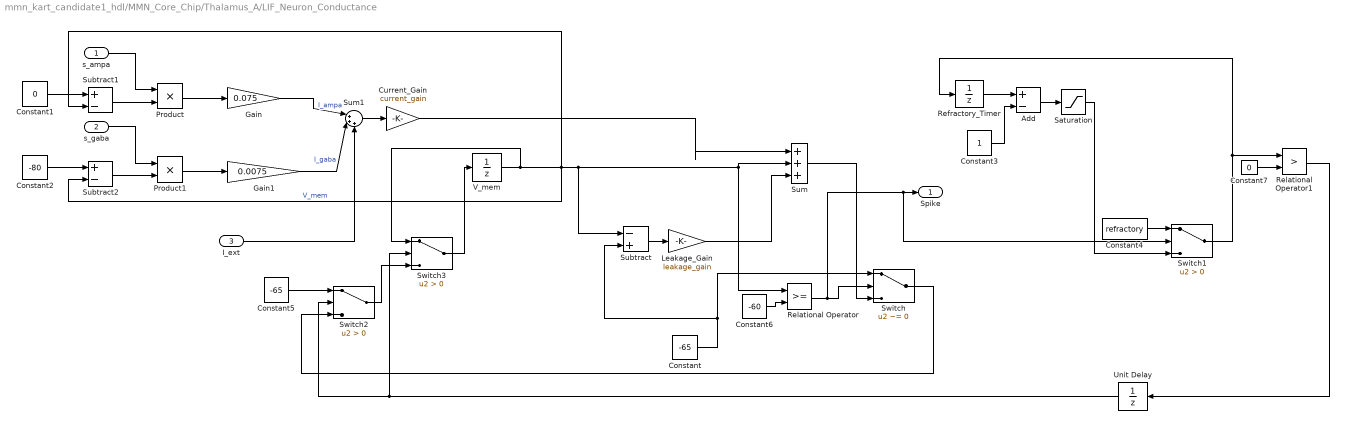
== system mmn_kart_candidate1_hdl/MMN_Core_Chip/Thalamus_A/LIF_Neuron_Conductance ==
  s_ampa : Inport  OutDataTypeStr=fixdt(1,24,8)
  s_gaba : Inport  Port=2  OutDataTypeStr=fixdt(1,24,8)
  I_ext : Inport  Port=3  OutDataTypeStr=fixdt(1,24,8)
  Add : Sum  Inputs=+-  OutDataTypeStr=fixdt(1,32,8)  AccumDataTypeStr=fixdt(1,32,8)  SaturateOnIntegerOverflow=on
  Constant : Constant  Value=-65  OutDataTypeStr=fixdt(1,32,8)
  Constant1 : Constant  Value=0  OutDataTypeStr=fixdt(1,32,8)
  Constant2 : Constant  Value=-80  OutDataTypeStr=fixdt(1,32,8)
  Constant3 : Constant  OutDataTypeStr=fixdt(1,32,8)
  Constant4 : Constant  Value=refractory  OutDataTypeStr=fixdt(1,32,8)
  Constant5 : Constant  Value=-65  OutDataTypeStr=fixdt(1,32,8)
  Constant6 : Constant  Value=-60  OutDataTypeStr=fixdt(1,32,8)
  Constant7 : Constant  Value=0  OutDataTypeStr=fixdt(1,32,8)
  Current_Gain : Gain  Gain=current_gain  ParamDataTypeStr=fixdt(1,24,20)  OutDataTypeStr=fixdt(1,32,8)  SaturateOnIntegerOverflow=on
  Gain : Gain  Gain=0.075  ParamDataTypeStr=fixdt(1,24,20)  OutDataTypeStr=fixdt(1,32,8)  SaturateOnIntegerOverflow=on
  Gain1 : Gain  Gain=0.0075  ParamDataTypeStr=fixdt(1,24,20)  OutDataTypeStr=fixdt(1,32,8)  SaturateOnIntegerOverflow=on
  Leakage_Gain : Gain  Gain=leakage_gain  ParamDataTypeStr=fixdt(1,24,20)  OutDataTypeStr=fixdt(1,32,8)  SaturateOnIntegerOverflow=on
  Product : Product  OutDataTypeStr=fixdt(1,32,8)  SaturateOnIntegerOverflow=on
  Product1 : Product  OutDataTypeStr=fixdt(1,32,8)  SaturateOnIntegerOverflow=on
  Refractory_Timer : UnitDelay  SampleTime=-1  HasFrameUpgradeWarning=on
  Relational Operator : RelationalOperator  OutDataTypeStr=boolean  RndMeth=Simplest  InputSameDT=off
  Relational Operator1 : RelationalOperator  Operator=>  OutDataTypeStr=boolean  RndMeth=Simplest  InputSameDT=off
  Saturation : Saturate  UpperLimit=40  LowerLimit=0  OutDataTypeStr=fixdt(1,32,8)
  Subtract : Sum  Inputs=-+  OutDataTypeStr=fixdt(1,32,8)  AccumDataTypeStr=fixdt(1,32,8)  SaturateOnIntegerOverflow=on
  Subtract1 : Sum  Inputs=+-  OutDataTypeStr=fixdt(1,32,8)  AccumDataTypeStr=fixdt(1,32,8)  SaturateOnIntegerOverflow=on
  Subtract2 : Sum  Inputs=+-  OutDataTypeStr=fixdt(1,32,8)  AccumDataTypeStr=fixdt(1,32,8)  SaturateOnIntegerOverflow=on
  Sum : Sum  Inputs=|+++  OutDataTypeStr=fixdt(1,32,8)  AccumDataTypeStr=fixdt(1,32,8)  SaturateOnIntegerOverflow=on
  Sum1 : Sum  Inputs=|+++  OutDataTypeStr=fixdt(1,32,8)  AccumDataTypeStr=fixdt(1,32,8)  SaturateOnIntegerOverflow=on
  Switch : Switch  Criteria=u2 ~= 0  OutDataTypeStr=fixdt(1,32,8)  InputSameDT=off
  Switch1 : Switch  Criteria=u2 > Threshold  OutDataTypeStr=fixdt(1,32,8)  InputSameDT=off
  Switch2 : Switch  Criteria=u2 > Threshold  OutDataTypeStr=fixdt(1,32,8)  InputSameDT=off
  Switch3 : Switch  Criteria=u2 > Threshold  OutDataTypeStr=fixdt(1,32,8)  InputSameDT=off
  Unit Delay : UnitDelay  SampleTime=-1  HasFrameUpgradeWarning=on
  V_mem : UnitDelay  InitialCondition=-65* ones(10, 1)  SampleTime=-1  HasFrameUpgradeWarning=on
  Spike : Outport  OutDataTypeStr=boolean
  wires:
  Gain1/1 -> Sum1/2  "I_gaba"
  Leakage_Gain/1 -> Sum/3
  Subtract2/1 -> Product1/2
  Relational Operator/1 -> Switch1/2, Spike/1, Switch/2
  Constant1/1 -> Subtract1/1
  Constant/1 -> Subtract/2, Switch/1
  s_ampa/1 -> Product/1
  Product/1 -> Gain/1
  Subtract1/1 -> Product/2
  Gain/1 -> Sum1/1  "I_ampa"
  Switch/1 -> Switch2/3
  Product1/1 -> Gain1/1
  s_gaba/1 -> Product1/1
  Subtract/1 -> Leakage_Gain/1
  Constant2/1 -> Subtract2/1
  Current_Gain/1 -> Sum/1
  Sum/1 -> Switch/3
  Sum1/1 -> Current_Gain/1
  I_ext/1 -> Sum1/3
  Refractory_Timer/1 -> Add/1
  Constant3/1 -> Add/2
  Add/1 -> Saturation/1
  Constant4/1 -> Switch1/1
  Saturation/1 -> Switch1/3
  Switch1/1 -> Refractory_Timer/1, Relational Operator1/1
  Relational Operator1/1 -> Unit Delay/1
  Constant5/1 -> Switch2/1
  Constant6/1 -> Relational Operator/2
  Constant7/1 -> Relational Operator1/2
  Unit Delay/1 -> Switch3/2, Switch2/2
  V_mem/1 -> Switch3/1, Subtract1/2, Subtract2/2, Relational Operator/1, Sum/2, Subtract/1  "V_mem"
  Switch2/1 -> Switch3/3
  Switch3/1 -> V_mem/1

== matlab function mmn_kart_candidate1_hdl/MMN_Core_Chip/MATLAB Function ==
  data: spikes_pre input; I_syn output; spikes_post input
function I_syn = STDP_Engine(spikes_pre, spikes_post)
%#codegen

T = fimath('RoundingMethod', 'Nearest', ...
           'OverflowAction', 'Saturate', ...
           'ProductMode', 'SpecifyPrecision', ...
           'ProductWordLength', 32, ...
           'ProductFractionLength', 20, ...
           'SumMode', 'SpecifyPrecision', ...
           'SumWordLength', 32, ...
           'SumFractionLength', 20);

type_w = numerictype(1, 16, 8);
type_t = numerictype(1, 18, 17);

I_syn = fi(zeros(10, 1), type_w, T);

persistent weights
persistent trace_pre
persistent trace_post

PARAM_decay_pre  = fi(0.99584, type_t, T);
PARAM_decay_post = fi(0.99792, type_t, T);
PARAM_A_plus     = fi(0.02, type_t, T);
PARAM_A_minus    = fi(0.03, type_t, T);
PARAM_w_min      = fi(0.01, type_w, T);
PARAM_w_max      = fi(10.0, type_w, T);
PARAM_w_init     = fi(0.4, type_w, T);
PARAM_ltd_gain   = fi(2.0, type_w, T);

if isempty(weights)
    weights    = repmat(PARAM_w_init, 10, 100);
    trace_pre  = fi(zeros(100, 1), type_t, T);
    trace_post = fi(zeros(10, 1), type_t, T);
end

PARAM_trace_pre_eps = fi(0.0027, type_t, T);
for j = 1:100
    tmp_pre = trace_pre(j) * PARAM_decay_pre;
    trace_pre(j) = fi(tmp_pre, type_t, T);

    if trace_pre(j) < PARAM_trace_pre_eps
        trace_pre(j) = fi(0, type_t, T);
    end
end

PARAM_trace_post_eps = fi(-0.0161, type_t, T);
for i = 1:10
    tmp_post = trace_post(i) * PARAM_decay_post;
    trace_post(i) = fi(tmp_post, type_t, T);

    if trace_post(i) > PARAM_trace_post_eps
        trace_post(i) = fi(0, type_t, T);
    end
end

coder.unroll(false);
for r = 1:10
    toplam = fi(0.0, type_w, T);

    for c = 1:100
        w_val = weights(r, c);

        if spikes_post(r) ~= 0
            delta_LTP = fi(trace_pre(c), type_w, T);
            w_val = fi(w_val + delta_LTP, type_w, T);
        end

        if spikes_pre(c) ~= 0
            delta_LTD = fi(PARAM_ltd_gain * trace_post(r), type_w, T);
            w_val = fi(w_val + delta_LTD, type_w, T);
        end

        if w_val > PARAM_w_max
            w_val = PARAM_w_max;
        elseif w_val < PARAM_w_min
            w_val = PARAM_w_min;
        end

        weights(r, c) = w_val;

        if spikes_pre(c) ~= 0
            toplam = fi(toplam + w_val, type_w, T);
        end
    end

    I_syn(r) = toplam;
end

for j = 1:100
    if spikes_pre(j) ~= 0
        trace_pre(j) = fi(trace_pre(j) + PARAM_A_plus, type_t, T);
    end
end

for i = 1:10
    if spikes_post(i) ~= 0
        trace_post(i) = fi(trace_post(i) - PARAM_A_minus, type_t, T);
    end
end
end
